simulink model "newQuatLib"  (R2015a)
settings: Solver=ode45  StartTime=0.0  StopTime=10.0  RelTol=1e-3
undefined symbols (not defined in the file): randquatiso
libraries: simulink x1
(part 2 of 2)

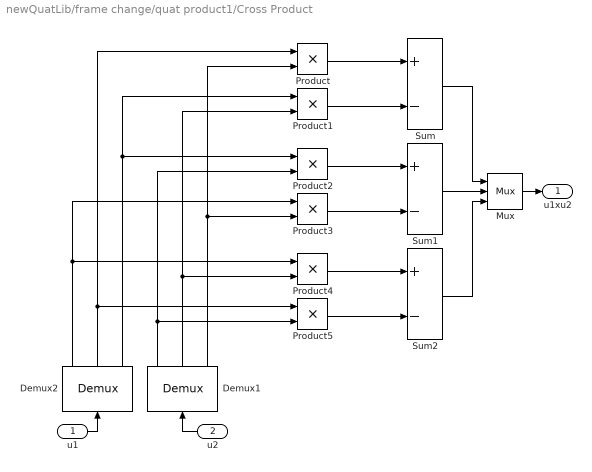
== system newQuatLib/frame change/quat product1/Cross Product ==
  u1 : Inport
  u2 : Inport  Port=2
  Demux1 : Demux  Outputs=3
  Demux2 : Demux  Outputs=3
  Mux : Mux  Inputs=3
  Product{,1..5} (6 alike) : Product  SaturateOnIntegerOverflow=on  RndMeth=Zero  InputSameDT=on  OutDataTypeStr=Inherit: Same as first input
  Sum : Sum  Inputs=+-  SaturateOnIntegerOverflow=on  InputSameDT=on  OutDataTypeStr=Inherit: Same as first input
  Sum1 : Sum  Inputs=+-  SaturateOnIntegerOverflow=on  InputSameDT=on  OutDataTypeStr=Inherit: Same as first input
  Sum2 : Sum  Inputs=+-  SaturateOnIntegerOverflow=on  InputSameDT=on  OutDataTypeStr=Inherit: Same as first input
  u1xu2 : Outport  InitialOutput=0
  wires:
  Sum2/1 -> Mux/3
  Sum1/1 -> Mux/2
  Sum/1 -> Mux/1
  Demux1/1 -> Product5/2, Product2/2
  Demux2/2 -> Product5/1, Product/1
  Demux1/2 -> Product4/2, Product1/2
  Demux2/1 -> Product4/1, Product3/1
  Demux1/3 -> Product3/2, Product/2
  Demux2/3 -> Product2/1, Product1/1
  Product5/1 -> Sum2/2
  Product4/1 -> Sum2/1
  Product3/1 -> Sum1/2
  Product2/1 -> Sum1/1
  Product1/1 -> Sum/2
  Product/1 -> Sum/1
  Mux/1 -> u1xu2/1
  u1/1 -> Demux2/1
  u2/1 -> Demux1/1

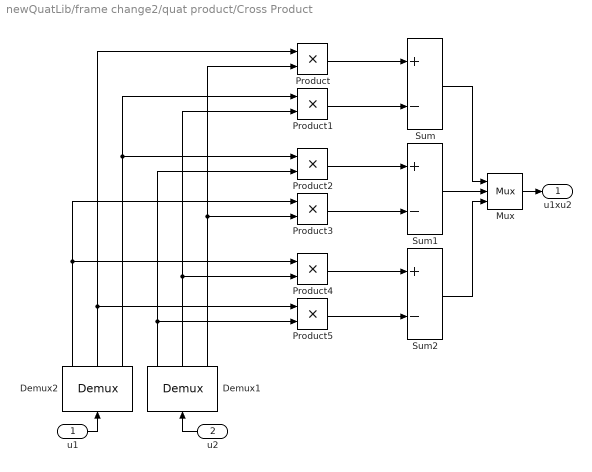
== system newQuatLib/frame change2/quat product/Cross Product ==
  u1 : Inport
  u2 : Inport  Port=2
  Demux1 : Demux  Outputs=3
  Demux2 : Demux  Outputs=3
  Mux : Mux  Inputs=3
  Product{,1..5} (6 alike) : Product  SaturateOnIntegerOverflow=on  RndMeth=Zero  InputSameDT=on  OutDataTypeStr=Inherit: Same as first input
  Sum : Sum  Inputs=+-  SaturateOnIntegerOverflow=on  InputSameDT=on  OutDataTypeStr=Inherit: Same as first input
  Sum1 : Sum  Inputs=+-  SaturateOnIntegerOverflow=on  InputSameDT=on  OutDataTypeStr=Inherit: Same as first input
  Sum2 : Sum  Inputs=+-  SaturateOnIntegerOverflow=on  InputSameDT=on  OutDataTypeStr=Inherit: Same as first input
  u1xu2 : Outport  InitialOutput=0
  wires:
  Sum2/1 -> Mux/3
  Sum1/1 -> Mux/2
  Sum/1 -> Mux/1
  Demux1/1 -> Product5/2, Product2/2
  Demux2/2 -> Product5/1, Product/1
  Demux1/2 -> Product4/2, Product1/2
  Demux2/1 -> Product4/1, Product3/1
  Demux1/3 -> Product3/2, Product/2
  Demux2/3 -> Product2/1, Product1/1
  Product5/1 -> Sum2/2
  Product4/1 -> Sum2/1
  Product3/1 -> Sum1/2
  Product2/1 -> Sum1/1
  Product1/1 -> Sum/2
  Product/1 -> Sum/1
  Mux/1 -> u1xu2/1
  u1/1 -> Demux2/1
  u2/1 -> Demux1/1

== system newQuatLib/frame change2/quat product1/Cross Product ==
  u1 : Inport
  u2 : Inport  Port=2
  Demux1 : Demux  Outputs=3
  Demux2 : Demux  Outputs=3
  Mux : Mux  Inputs=3
  Product{,1..5} (6 alike) : Product  SaturateOnIntegerOverflow=on  RndMeth=Zero  InputSameDT=on  OutDataTypeStr=Inherit: Same as first input
  Sum : Sum  Inputs=+-  SaturateOnIntegerOverflow=on  InputSameDT=on  OutDataTypeStr=Inherit: Same as first input
  Sum1 : Sum  Inputs=+-  SaturateOnIntegerOverflow=on  InputSameDT=on  OutDataTypeStr=Inherit: Same as first input
  Sum2 : Sum  Inputs=+-  SaturateOnIntegerOverflow=on  InputSameDT=on  OutDataTypeStr=Inherit: Same as first input
  u1xu2 : Outport  InitialOutput=0
  wires:
  u2/1 -> Demux1/1
  u1/1 -> Demux2/1
  Mux/1 -> u1xu2/1
  Product/1 -> Sum/1
  Product1/1 -> Sum/2
  Product2/1 -> Sum1/1
  Product3/1 -> Sum1/2
  Product4/1 -> Sum2/1
  Product5/1 -> Sum2/2
  Demux2/3 -> Product1/1, Product2/1
  Demux1/3 -> Product/2, Product3/2
  Demux2/1 -> Product3/1, Product4/1
  Demux1/2 -> Product1/2, Product4/2
  Demux2/2 -> Product/1, Product5/1
  Demux1/1 -> Product2/2, Product5/2
  Sum/1 -> Mux/1
  Sum1/1 -> Mux/2
  Sum2/1 -> Mux/3

== system newQuatLib/qDot/quat product/Cross Product ==
  u1 : Inport
  u2 : Inport  Port=2
  Demux1 : Demux  Outputs=3
  Demux2 : Demux  Outputs=3
  Mux : Mux  Inputs=3
  Product{,1..5} (6 alike) : Product  SaturateOnIntegerOverflow=on  RndMeth=Zero  InputSameDT=on  OutDataTypeStr=Inherit: Same as first input
  Sum : Sum  Inputs=+-  SaturateOnIntegerOverflow=on  InputSameDT=on  OutDataTypeStr=Inherit: Same as first input
  Sum1 : Sum  Inputs=+-  SaturateOnIntegerOverflow=on  InputSameDT=on  OutDataTypeStr=Inherit: Same as first input
  Sum2 : Sum  Inputs=+-  SaturateOnIntegerOverflow=on  InputSameDT=on  OutDataTypeStr=Inherit: Same as first input
  u1xu2 : Outport  InitialOutput=0
  wires:
  Sum2/1 -> Mux/3
  Sum1/1 -> Mux/2
  Sum/1 -> Mux/1
  Demux1/1 -> Product5/2, Product2/2
  Demux2/2 -> Product5/1, Product/1
  Demux1/2 -> Product4/2, Product1/2
  Demux2/1 -> Product4/1, Product3/1
  Demux1/3 -> Product3/2, Product/2
  Demux2/3 -> Product2/1, Product1/1
  Product5/1 -> Sum2/2
  Product4/1 -> Sum2/1
  Product3/1 -> Sum1/2
  Product2/1 -> Sum1/1
  Product1/1 -> Sum/2
  Product/1 -> Sum/1
  Mux/1 -> u1xu2/1
  u1/1 -> Demux2/1
  u2/1 -> Demux1/1

== system newQuatLib/quat2W/quat product/Cross Product ==
  u1 : Inport
  u2 : Inport  Port=2
  Demux1 : Demux  Outputs=3
  Demux2 : Demux  Outputs=3
  Mux : Mux  Inputs=3
  Product{,1..5} (6 alike) : Product  SaturateOnIntegerOverflow=on  RndMeth=Zero  InputSameDT=on  OutDataTypeStr=Inherit: Same as first input
  Sum : Sum  Inputs=+-  SaturateOnIntegerOverflow=on  InputSameDT=on  OutDataTypeStr=Inherit: Same as first input
  Sum1 : Sum  Inputs=+-  SaturateOnIntegerOverflow=on  InputSameDT=on  OutDataTypeStr=Inherit: Same as first input
  Sum2 : Sum  Inputs=+-  SaturateOnIntegerOverflow=on  InputSameDT=on  OutDataTypeStr=Inherit: Same as first input
  u1xu2 : Outport  InitialOutput=0
  wires:
  u2/1 -> Demux1/1
  u1/1 -> Demux2/1
  Mux/1 -> u1xu2/1
  Product/1 -> Sum/1
  Product1/1 -> Sum/2
  Product2/1 -> Sum1/1
  Product3/1 -> Sum1/2
  Product4/1 -> Sum2/1
  Product5/1 -> Sum2/2
  Demux2/3 -> Product1/1, Product2/1
  Demux1/3 -> Product/2, Product3/2
  Demux2/1 -> Product3/1, Product4/1
  Demux1/2 -> Product1/2, Product4/2
  Demux2/2 -> Product/1, Product5/1
  Demux1/1 -> Product2/2, Product5/2
  Sum/1 -> Mux/1
  Sum1/1 -> Mux/2
  Sum2/1 -> Mux/3

== system newQuatLib/quat2W/unwrap quat/get index of (first) largest component ==
  q : Inport
  Abs : Abs
  Relational Operator : RelationalOperator  Operator===
  discriminate : Gain  Gain=[1 2 3 4]
  double : DataTypeConversion  OutDataTypeStr=double
  find : MinMax  Function=max
  max : MinMax  Function=max
  idx(max(abs(q)) : Outport
  wires:
  double/1 -> discriminate/1
  discriminate/1 -> find/1
  q/1 -> Abs/1
  Abs/1 -> max/1, Relational Operator/1
  max/1 -> Relational Operator/2
  Relational Operator/1 -> double/1  "1 for the greatest component(s)"
  find/1 -> idx(max(abs(q))/1  "index of first greatest component"

== system newQuatLib/random isotropic quaternion/Normalization/Norm ==
  X : Inport
  Dot Product1 : DotProduct  InputSameDT=on  OutDataTypeStr=Inherit: Inherit via internal rule
  Math Function : Math  Operator=sqrt  SaturateOnIntegerOverflow=on
  ||X|| : Outport  InitialOutput=0
  wires:
  Math Function/1 -> ||X||/1
  Dot Product1/1 -> Math Function/1
  X/1 -> Dot Product1/2, Dot Product1/1

== system newQuatLib/vects2frame/Normalization/Norm ==
  X : Inport
  Dot Product1 : DotProduct  InputSameDT=on  OutDataTypeStr=Inherit: Inherit via internal rule
  Math Function : Math  Operator=sqrt  SaturateOnIntegerOverflow=on
  ||X|| : Outport  InitialOutput=0
  wires:
  X/1 -> Dot Product1/1, Dot Product1/2
  Dot Product1/1 -> Math Function/1
  Math Function/1 -> ||X||/1

== system newQuatLib/vects2frame/Normalization1/Norm ==
  X : Inport
  Dot Product1 : DotProduct  InputSameDT=on  OutDataTypeStr=Inherit: Inherit via internal rule
  Math Function : Math  Operator=sqrt  SaturateOnIntegerOverflow=on
  ||X|| : Outport  InitialOutput=0
  wires:
  Math Function/1 -> ||X||/1
  Dot Product1/1 -> Math Function/1
  X/1 -> Dot Product1/2, Dot Product1/1

== matlab function newQuatLib/interpolate between 2 quats/MATLAB Function ==
  data: q1 input; qi output; q2 input; k input
function qi = slerp (q1, q2, k)

eps = 0.001;

if k==0 % saving calculation time -> where qm=qi
    qi=q1;
    
elseif k==1 % saving calculation time -> where qm=qn
    qi=q2;
    
else

    C=q1'*q2;                  % Calculating the angle beteen the unit quaternions by dot product

    teta=acos(C);

        if (1 - C) <= eps % if angle teta is close by epsilon to 0 degrees -> calculate by linear interpolation
            qi=q1*(1-k)+q2*k; % avoiding divisions by number close to 0

        elseif (1 + C) <= eps % when teta is close by epsilon to 180 degrees the result is undefined -> no shortest direction to rotate
            q2(1) = q1(4); q2(2) = -q1(3); q2(3)= q1(2); q2(4) = -q1(1); % rotating one of the unit quaternions by 90 degrees -> q2
            qi=q1*(sin((1-k)*(pi/2)))+q2*sin(k*(pi/2));

        else
            qi=q1*(sin((1-k)*teta))/sin(teta)+q2*sin(k*teta)/sin(teta);
        end
end

== matlab function newQuatLib/frame2quat/MATLAB Function ==
  data: xB input; qA2B output; yB input; zB input
function qA2B = frame2quat(xB,yB,zB)
%#codegen

A = zeros(1,4);
T = [xB(:),yB(:),zB(:)];
qA2B = zeros(4,1);

A(1) =  T(1,1) + T(2,2) + T(3,3);
A(2) =  T(1,1) - T(2,2) - T(3,3);
A(3) = -T(1,1) + T(2,2) - T(3,3);
A(4) = -T(1,1) - T(2,2) + T(3,3);

[~,idx] = max(A);

switch idx
    case 1
        qA2B(1) = 0.5*sqrt(1+A(1));
        D = 1/(4*qA2B(1));
        qA2B(2) = (T(3,2)-T(2,3))*D;
        qA2B(3) = (T(1,3)-T(3,1))*D;
        qA2B(4) = (T(2,1)-T(1,2))*D;
    case 2
        qA2B(2) = 0.5*sqrt(1+A(2));
        D = 1/(4*qA2B(2));
        qA2B(3) = (T(2,1)+T(1,2))*D;
        qA2B(4) = (T(1,3)+T(3,1))*D;
        qA2B(1) = (T(3,2)-T(2,3))*D;
    case 3
        qA2B(3) = 0.5*sqrt(1+A(3));
        D = 1/(4*qA2B(3));
        qA2B(4) = (T(3,2)+T(2,3))*D;
        qA2B(1) = (T(1,3)-T(3,1))*D;
        qA2B(2) = (T(2,1)+T(1,2))*D;
    case 4
        qA2B(4) = 0.5*sqrt(1+A(4));
        D = 1/(4*qA2B(4));
        qA2B(1) = (T(2,1)-T(1,2))*D;
        qA2B(2) = (T(1,3)+T(3,1))*D;
        qA2B(3) = (T(3,2)+T(2,3))*D;
end % switch
